simulink model "Pacejka2"  (R2020a)
settings: Solver=VariableStepAuto  StartTime=0.0  StopTime=10.0  RelTol=1e-3
undefined symbols (not defined in the file or in its folder): a0, a1, a10, a11, a12, a13, a14, a15, a16, a17, a2, a3, a4, a5, a6, a7, a8, a9, camber
settings Model: Creator=carmelo  LastModifiedBy=carmelo

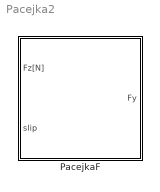
== system Pacejka2 ==
  PacejkaF : Subsystem

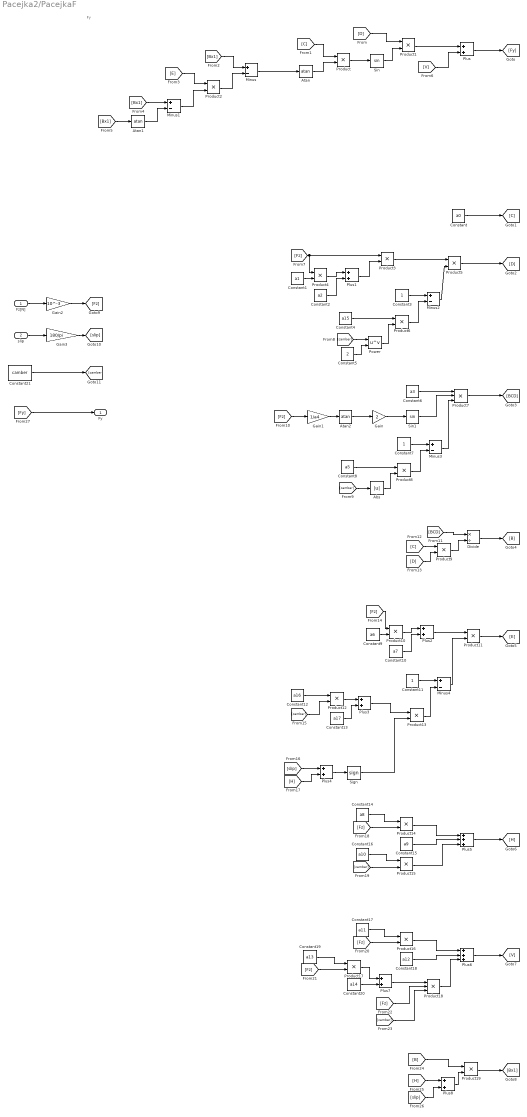
== system Pacejka2/PacejkaF ==
  note: Fy
  Fz[N] : Inport  Unit=N
  slip : Inport  Port=2  Unit=rad
  Abs : Abs
  Atan : Trigonometry  Operator=atan
  Atan1 : Trigonometry  Operator=atan
  Atan2 : Trigonometry  Operator=atan
  Constant : Constant  Value=a0
  Constant1 : Constant  Value=a1
  Constant10 : Constant  Value=a7
  Constant11 : Constant
  Constant12 : Constant  Value=a16
  Constant13 : Constant  Value=a17
  Constant14 : Constant  Value=a8
  Constant15 : Constant  Value=a9
  Constant16 : Constant  Value=a10
  Constant17 : Constant  Value=a11
  Constant18 : Constant  Value=a12
  Constant19 : Constant  Value=a13
  Constant2 : Constant  Value=a2
  Constant20 : Constant  Value=a14
  Constant21 : Constant  Value=camber
  Constant3 : Constant
  Constant4 : Constant  Value=a15
  Constant5 : Constant  Value=2
  Constant6 : Constant  Value=a3
  Constant7 : Constant
  Constant8 : Constant  Value=a5
  Constant9 : Constant  Value=a6
  Divide : Product  Inputs=*/
  Gain : Gain  Gain=2
  Gain1 : Gain  Gain=1/a4
  Gain2 : Gain  Gain=10^-3
  Gain3 : Gain  Gain=180/pi
  Minus{,1..4} (5 alike) : Sum  Inputs=+-
  Plus{,1..4,7..8} (7 alike) : Sum
  Plus5 : Sum  Inputs=+++
  Plus6 : Sum  Inputs=+++
  Power : Math  Operator=pow  SaturateOnIntegerOverflow=on
  Product{,1..6,8..17,19} (18 alike) : Product
  Product18 : Product  Inputs=3
  Product7 : Product  Inputs=3
  Sign : Signum  ZeroCross=off
  Sin : Trigonometry
  Sin1 : Trigonometry
  Fy : Outport  Unit=N
  wires:
  Product/1 -> Sin/1
  Product2/1 -> Minus/2
  slip/1 -> Gain3/1
  Product3/1 -> Product5/1
  Minus3/1 -> Product7/3
  Product15/1 -> Plus5/3
  Abs/1 -> Product8/2
  Constant14/1 -> Product14/1
  Gain2/1 -> [Fz]
  Constant/1 -> [C]
  Atan/1 -> Product/2
  [Fy] -> Fy/1
  Gain1/1 -> Atan2/1
  [B] -> Product19/1
  [Fz] -> Product14/2
  [Bx1] -> Minus/1
  [Fz] -> Product18/2
  Gain3/1 -> [slip]
  Gain/1 -> Sin1/1
  [Fz] -> Product10/1
  [slip] -> Plus8/2
  Plus6/1 -> [V]
  Plus2/1 -> Product11/1
  [D] -> Product1/1
  Plus5/1 -> [H]
  Minus4/1 -> Product11/2
  Minus/1 -> Atan/1
  Constant6/1 -> Product7/1
  [camber] -> Product12/2
  [V] -> Plus/2
  Product6/1 -> Minus2/2
  [C] -> Product/1
  Product19/1 -> [Bx1]
  Fz[N]/1 -> Gain2/1
  Constant21/1 -> [camber]
  Product16/1 -> Plus6/1
  Constant7/1 -> Minus3/1
  [Fz] -> Product17/2
  Product14/1 -> Plus5/1
  [BCD] -> Divide/1
  Constant20/1 -> Plus7/2
  Sin/1 -> Product1/2
  Sign/1 -> Product13/2
  Product7/1 -> [BCD]
  [camber] -> Abs/1
  Plus7/1 -> Product18/1
  Constant15/1 -> Plus5/2
  Product12/1 -> Plus3/1
  Constant18/1 -> Plus6/2
  Product11/1 -> [E]
  [Bx1] -> Minus1/1
  [Fz] -> Gain1/1
  Plus/1 -> [Fy]
  Divide/1 -> [B]
  Constant16/1 -> Product15/1
  [H] -> Plus8/1
  Atan2/1 -> Gain/1
  Plus3/1 -> Product13/1
  Constant17/1 -> Product16/1
  Product17/1 -> Plus7/1
  Plus1/1 -> Product3/2
  Product18/1 -> Plus6/3
  Constant13/1 -> Plus3/2
  Product10/1 -> Plus2/1
  Sin1/1 -> Product7/2
  [Fz] -> Product16/2
  [Bx1] -> Atan1/1
  Constant2/1 -> Plus1/2
  Constant3/1 -> Minus2/1
  [camber] -> Power/1
  [camber] -> Product18/3
  Minus1/1 -> Product2/2
  [C] -> Product9/1
  [camber] -> Product15/2
  [Fz] -> Product4/1, Product3/1
  Power/1 -> Product6/2
  Constant9/1 -> Product10/2
  [D] -> Product9/2
  Constant4/1 -> Product6/1
  Atan1/1 -> Minus1/2
  Constant19/1 -> Product17/1
  Product13/1 -> Minus4/2
  Product1/1 -> Plus/1
  Product4/1 -> Plus1/1
  Constant5/1 -> Power/2
  Product5/1 -> [D]
  Plus8/1 -> Product19/2
  Minus2/1 -> Product5/2
  [E] -> Product2/1
  Constant1/1 -> Product4/2
  Constant11/1 -> Minus4/1
  Constant10/1 -> Plus2/2
  Constant12/1 -> Product12/1
  Product8/1 -> Minus3/2
  Constant8/1 -> Product8/1
  Product9/1 -> Divide/2
  [H] -> Plus4/2
  Plus4/1 -> Sign/1
  [slip] -> Plus4/1
